simulink model "SG__MDL_IO344"  (R2020a)
settings: Solver=FixedStepAuto  StartTime=0.0  StopTime=Inf  RelTol=1e-3  EnableMultiTasking=on
model workspace (MAT data in the model file):
  a = 0.28
  ff = 1200
  fi = 150
  tmax = 40
libraries: dspfdesign x4, slrtlib x3, simulink x2, SG_library x1, dspsrcs4 x1
settings Model: SimulationMode=external  Creator=padlewsk  LastModifiedBy=padlewsk
settings SolverCC: ConcurrentTasks=on  AutoInsertRateTranBlk=on
settings DataIOCC: SaveFormat=StructureWithTime
settings OptimizationCC: BlockReduction=off  OptimizeBlockIOStorage=off
settings DebuggingCC: SFMachineParentedDataDiag=error
settings HardwareCC: ProdBitPerPointer=32  ProdBitPerSizeT=32  ProdBitPerPtrDiffT=32  ProdLargestAtomicFloat=None  ProdWordSize=32  ProdLongLongMode=on  ProdHWDeviceType=Generic->32-bit x86 compatible
settings RTWCC: Description=Simulink Real-Time  SystemTargetFile=slrt.tlc  TemplateMakefile=slrt_default_tmf  CodeExecutionProfiling=on  RTWCompilerOptimization=on
settings SimulinkRealTimeCC: SupportVariableSizeSignals=on  xPCConcurrentTasks=on

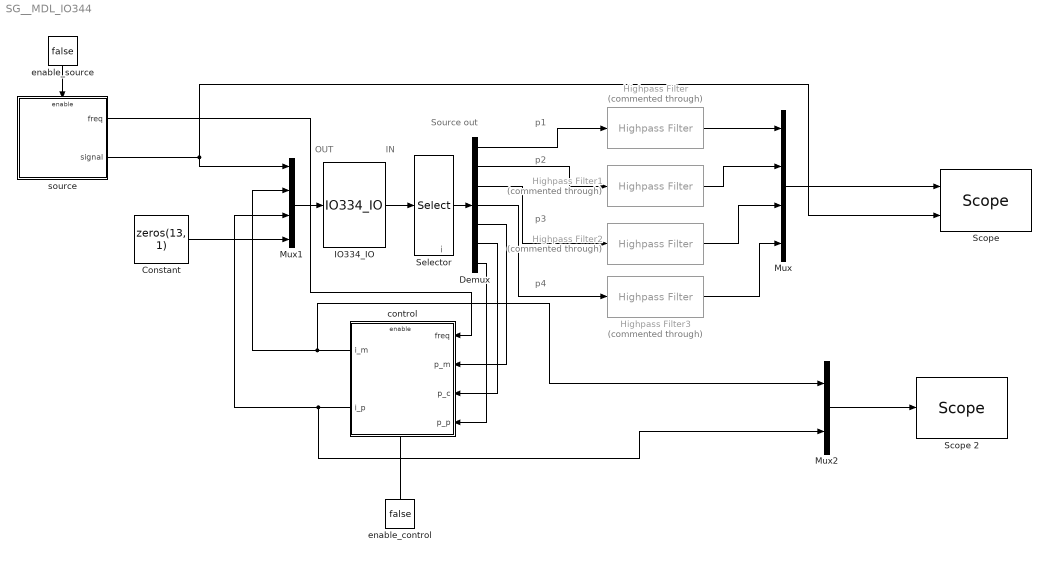
== system SG__MDL_IO344 ==
  note: p2
  note: i
  note: p3
  note: p1
  note: Source out
  note: IN
  note: OUT
  note: p4
  Constant : Constant  Value=zeros(13, 1)  SampleTime=-1
  Demux : Demux  Outputs=7
  Highpass Filter : dspfdesign/Highpass Filter  Commented=through  FilterType=IIR  DesignForMinimumOrder=off  FilterOrder=4  StopbandFrequency=8e3  PassbandFrequency=5  StopbandAttenuation=80  PassbandRipple=0.1  InheritSampleRate=off  SampleRate=65536  SimulateUsing=Interpreted execution  roundingMode=Floor  coeffsDataTypeStr=fixdt(1,16)
  Highpass Filter1 : dspfdesign/Highpass Filter  Commented=through  FilterType=IIR  DesignForMinimumOrder=off  FilterOrder=4  StopbandFrequency=8e3  PassbandFrequency=5  StopbandAttenuation=80  PassbandRipple=0.1  InheritSampleRate=off  SampleRate=65536  SimulateUsing=Interpreted execution  roundingMode=Floor  coeffsDataTypeStr=fixdt(1,16)
  Highpass Filter2 : dspfdesign/Highpass Filter  Commented=through  FilterType=IIR  DesignForMinimumOrder=off  FilterOrder=4  StopbandFrequency=8e3  PassbandFrequency=5  StopbandAttenuation=80  PassbandRipple=0.1  InheritSampleRate=off  SampleRate=65536  SimulateUsing=Interpreted execution  roundingMode=Floor  coeffsDataTypeStr=fixdt(1,16)
  Highpass Filter3 : dspfdesign/Highpass Filter  Commented=through  FilterType=IIR  DesignForMinimumOrder=off  FilterOrder=4  StopbandFrequency=4  PassbandFrequency=5  StopbandAttenuation=80  PassbandRipple=0.1  InheritSampleRate=off  SampleRate=65536  SimulateUsing=Interpreted execution  roundingMode=Floor  coeffsDataTypeStr=fixdt(1,16)
  IO334_IO : SG_library/Built elements/IO334_IO  ts=1.5259e-05  OutputRange=Auto (same as ADC)
      settings: SourceProductName=Custom Speedgoat implementations
  Mux : Mux
  Mux1 : Mux
  Mux2 : Mux  Inputs=2
  "Scope " : slrtlib/Displays and Logging/Scope   scopeno=2  scopetype=Host  autostart=on  viewmode=Graphical redraw  formatstr='%15.6f'  grid=on  ylimits=[0,0]  nosamples=1000  noprepostsamples=0  interleave=1  triggermode=Signal triggering  triggersignal=1  trigsignalfromport=on  triggerlevel=0.001  triggerslope=Either  triggerscope=1  triggersample=0  filename=data.dat  mode=Lazy  writesize=512  autorestart=off  dynamicfilemode=off  maxwritefilesize=512*1024^2
  Scope 2 : slrtlib/Displays and Logging/Scope   scopeno=3  scopetype=Target  autostart=on  viewmode=Graphical redraw  formatstr='%15.6f'  grid=on  ylimits=[0 0]  nosamples=250  noprepostsamples=0  interleave=1  triggermode=FreeRun  triggersignal=1  trigsignalfromport=off  triggerlevel=0.45  triggerslope=Either  triggerscope=1  triggersample=0  filename=data.dat  mode=Lazy  writesize=512  autorestart=off  dynamicfilemode=off  maxwritefilesize=512*1024^2
  Selector : Selector  InputPortWidth=16  IndexOptions=Index vector (dialog)  Indices=1:7  OutputSizes=1
  control : Subsystem
  enable_control : Constant  Value=false  SampleTime=-1
  enable_source : Constant  Value=false  SampleTime=-1
  source : Subsystem  TreatAsAtomicUnit=on
  wires:
  enable_source/1 -> source/Enable
  Mux/1 -> "Scope "/1
  Highpass Filter2/1 -> Mux/3
  Demux/1 -> Highpass Filter/1
  Highpass Filter/1 -> Mux/1
  Demux/3 -> Highpass Filter2/1
  Highpass Filter1/1 -> Mux/2
  Demux/4 -> Highpass Filter3/1
  IO334_IO/1 -> Selector/1
  Constant/1 -> Mux1/4
  Selector/1 -> Demux/1
  Demux/2 -> Highpass Filter1/1
  Mux1/1 -> IO334_IO/1
  source/1(freq) -> control/1(freq)
  Demux/5 -> control/2(p_m)
  control/2(i_p) -> Mux2/2, Mux1/3
  enable_control/1 -> control/Enable
  Demux/7 -> control/4(p_p)
  Demux/6 -> control/3(p_c)
  source/2(signal) -> Mux1/1, "Scope "/2
  Mux2/1 -> Scope 2/1
  Highpass Filter3/1 -> Mux/4
  control/1(i_m) -> Mux2/1, Mux1/2

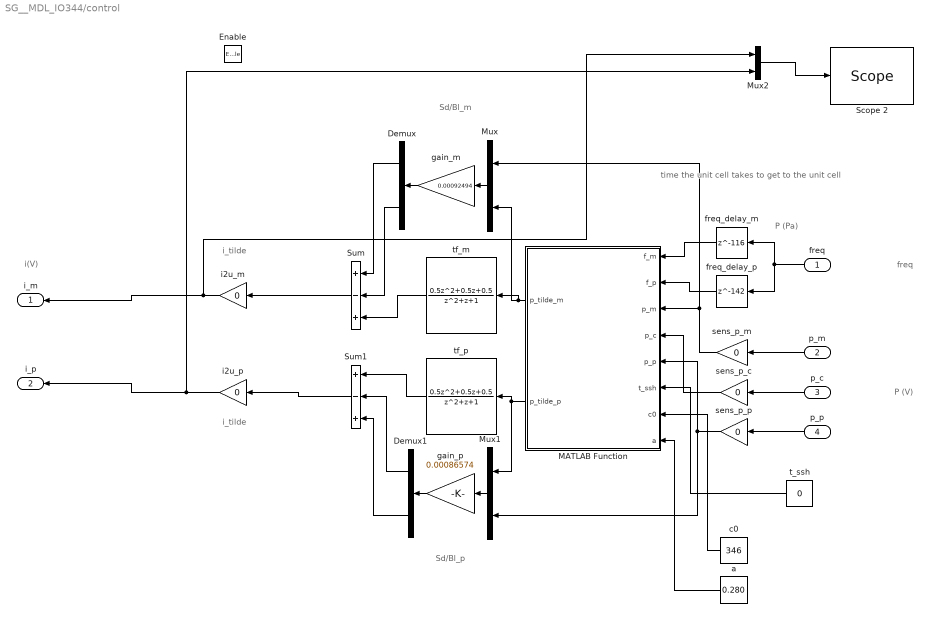
== system SG__MDL_IO344/control ==
  note: time the unit cell takes to get to the unit cell
  note: Sd/Bl_p
  note: P (Pa)
  note: P (V)
  note: i_tilde
  note: i(V)
  note: freq
  note: i_tilde
  note: Sd/Bl_m
  freq : Inport
  p_m : Inport  Port=2
  p_c : Inport  Port=3
  p_p : Inport  Port=4
  Enable : EnablePort
  Demux : Demux  Outputs=2
  Demux1 : Demux  Outputs=2
  MATLAB Function : MATLAB Function  TreatAsAtomicUnit=on
  Mux : Mux  Inputs=2
  Mux1 : Mux  Inputs=2
  Mux2 : Mux  Inputs=2
  Scope 2 : slrtlib/Displays and Logging/Scope   scopeno=1  scopetype=Target  autostart=on  viewmode=Graphical redraw  formatstr='%15.6f'  grid=on  ylimits=[0 0]  nosamples=250  noprepostsamples=0  interleave=1  triggermode=FreeRun  triggersignal=1  trigsignalfromport=off  triggerlevel=0.45  triggerslope=Either  triggerscope=1  triggersample=0  filename=data.dat  mode=Lazy  writesize=512  autorestart=off  dynamicfilemode=off  maxwritefilesize=512*1024^2
  Sum : Sum  Inputs=+-+
  Sum1 : Sum  Inputs=+-+
  a : Constant  Value=0.280
  c0 : Constant  Value=346
  freq_delay_m : Delay  DelayLength=116  InitialCondition=1
  freq_delay_p : Delay  DelayLength=142  InitialCondition=1
  gain_m : Gain  Gain=0.00092494
  gain_p : Gain  Gain=0.00086574
  i2u_m : Gain  Gain=0
  i2u_p : Gain  Gain=0
  sens_p_c : Gain  Gain=0
  sens_p_m : Gain  Gain=0
  sens_p_p : Gain  Gain=0
  t_ssh : Constant  Value=0
  tf_m : DiscreteTransferFcn  Numerator="[0.5         0.5         0.5]"  Denominator="[1  1  1]"
  tf_p : DiscreteTransferFcn  Numerator="[0.5         0.5         0.5]"  Denominator="[1  1  1]"
  i_m : Outport
  i_p : Outport  Port=2
  wires:
  p_m/1 -> sens_p_m/1
  sens_p_m/1 -> Mux/1, MATLAB Function/3(p_m)
  p_c/1 -> sens_p_c/1
  p_p/1 -> sens_p_p/1
  t_ssh/1 -> MATLAB Function/6(t_ssh)
  sens_p_c/1 -> MATLAB Function/4(p_c)
  sens_p_p/1 -> MATLAB Function/5(p_p), Mux1/2
  Demux1/1 -> Sum1/2
  Demux1/2 -> Sum1/3
  Demux/2 -> Sum/2
  Demux/1 -> Sum/1
  Mux/1 -> gain_m/1
  gain_m/1 -> Demux/1
  Mux1/1 -> gain_p/1
  gain_p/1 -> Demux1/1
  Mux2/1 -> Scope 2/1
  tf_m/1 -> Sum/3
  tf_p/1 -> Sum1/1
  freq/1 -> freq_delay_p/1, freq_delay_m/1
  i2u_p/1 -> Mux2/2, i_p/1
  freq_delay_m/1 -> MATLAB Function/1(f_m)
  i2u_m/1 -> Mux2/1, i_m/1
  freq_delay_p/1 -> MATLAB Function/2(f_p)
  c0/1 -> MATLAB Function/7(c0)
  a/1 -> MATLAB Function/8(a)
  MATLAB Function/2(p_tilde_p) -> Mux1/1, tf_p/1
  MATLAB Function/1(p_tilde_m) -> tf_m/1, Mux/2
  Sum/1 -> i2u_m/1
  Sum1/1 -> i2u_p/1

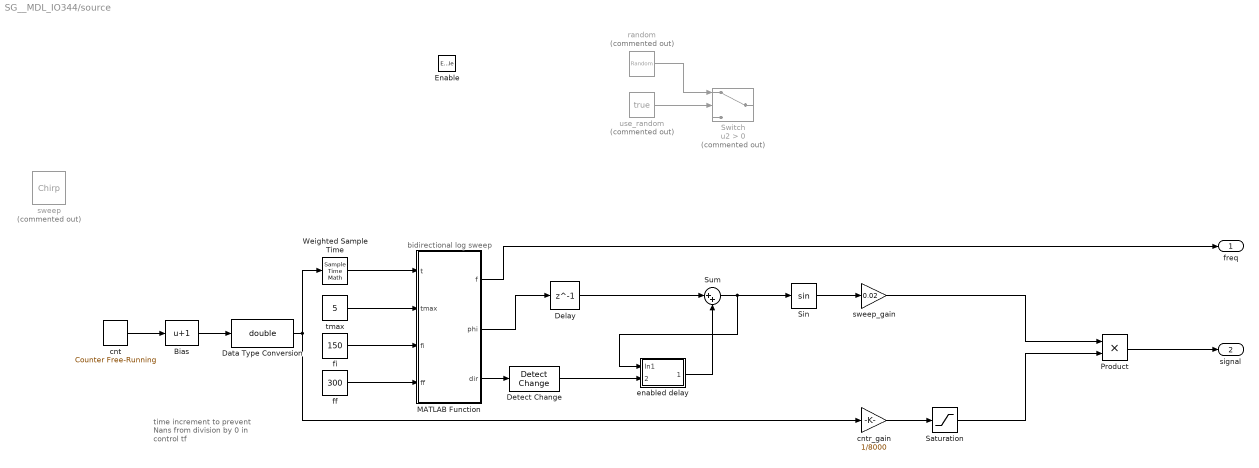
== system SG__MDL_IO344/source ==
  note: bidirectional log sweep
  note: time increment to prevent Nans from division by 0 in control tf
  Enable : EnablePort  StatesWhenEnabling=reset
  Bias : Bias  Bias=1
  Data Type Conversion : DataTypeConversion  OutDataTypeStr=double
  Delay : Delay  DelayLength=1
  Detect Change : simulink/Logic and Bit Operations/Detect Change  vinit=false  OutDataTypeStr=boolean
  MATLAB Function : MATLAB Function  TreatAsAtomicUnit=on
  Product : Product
  Saturation : Saturate  UpperLimit=1  LowerLimit=0
  Sin : Trigonometry
  Sum : Sum  Inputs=|++
  Switch : Switch  Commented=on  Criteria=u2 > Threshold
  Weighted Sample Time : SampleTimeMath  TsampMathOp=*
  cnt : simulink/Sources/Counter Free-Running  NumBits=32  tsamp=1.5259e-05
  cntr_gain : Gain  Gain=1/8000  ParamDataTypeStr=double
  enabled delay : Subsystem
  ff : Constant  Value=300
  fi : Constant  Value=150
  random : RandomNumber  Commented=on  Variance=0.5  SampleTime=3.5e-05
  sweep : dspsrcs4/Chirp  Commented=on  sweep=Logarithmic  mode=Bidirectional  f0=150  f1=1200  t1=10  Tsweep=20  phase=0  Ts=3.5e-05  spf=1  datatype=Double  OutputFrames=off
  sweep_gain : Gain  Gain=0.02
  tmax : Constant  Value=5
  use_random : Constant  Commented=on  Value=true  SampleTime=-1
  freq : Outport  OutputWhenDisabled=reset  InitialOutput=0  VectorParamsAs1DForOutWhenUnconnected=off
  signal : Outport  Port=2  OutputWhenDisabled=reset  InitialOutput=0  VectorParamsAs1DForOutWhenUnconnected=off
  wires:
  use_random/1 -> Switch/2
  random/1 -> Switch/1
  sweep_gain/1 -> Product/1
  cntr_gain/1 -> Saturation/1
  Product/1 -> signal/1
  MATLAB Function/2(phi) -> Delay/1
  Saturation/1 -> Product/2
  Weighted Sample Time/1 -> MATLAB Function/1(t)
  Data Type Conversion/1 -> cntr_gain/1, Weighted Sample Time/1
  MATLAB Function/1(f) -> freq/1
  Sin/1 -> sweep_gain/1
  MATLAB Function/3(dir) -> Detect Change/1
  Detect Change/1 -> enabled delay/2(enable)
  Delay/1 -> Sum/1
  enabled delay/1(Out1) -> Sum/2
  Sum/1 -> enabled delay/1(In1), Sin/1
  cnt/1 -> Bias/1
  Bias/1 -> Data Type Conversion/1
  ff/1 -> MATLAB Function/4(ff)
  tmax/1 -> MATLAB Function/2(tmax)
  fi/1 -> MATLAB Function/3(fi)

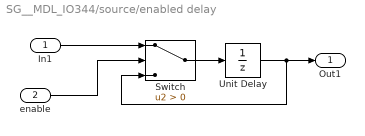
== system SG__MDL_IO344/source/enabled delay ==
  In1 : Inport
  enable : Inport  Port=2
  Switch : Switch  Criteria=u2 > Threshold
  Unit Delay : UnitDelay  SampleTime=-1  HasFrameUpgradeWarning=on
  Out1 : Outport
  wires:
  Unit Delay/1 -> Switch/3, Out1/1
  Switch/1 -> Unit Delay/1
  In1/1 -> Switch/1
  enable/1 -> Switch/2

== matlab function SG__MDL_IO344/control/MATLAB Function ==
  data: f_m input; f_p input; p_tilde_m output; p_m input; p_c input; p_p input; t_ssh input; p_tilde_p output; c0 input; a input
function [p_tilde_m, p_tilde_p] = p_tilde(f_m,f_p,p_m,p_c,p_p, t_ssh, c0, a)%frequency and pressure
% c0 and a are set as parameters and directly read from the workspace 
k_m = 2*pi*f_m/c0 %corresponding wave vector%%
k_p = 2*pi*f_p/c0 %corresponding wave vector%%

p_tilde_m = (p_m*sin(k_m*a*(t_ssh-1)/4) + p_c*sin(-k_m*a*t_ssh/4))/sin(-k_m*a/4) ;
p_tilde_p = (p_p*sin(-k_p*a*(t_ssh-1)/4) + p_c*sin(k_p*a*t_ssh/4))/sin(k_p*a/4) ;

%p_tilde_m = (p_c);
%p_tilde_p = (p_c);

== matlab function SG__MDL_IO344/source/MATLAB Function ==
  data: f output; t input; tmax input; phi output; dir output; fi input; ff input
function [f, phi, dir] = fcn(t, tmax, fi, ff)
%tmax is the time at which the maximum frequency is reached

t = mod(t, 2*tmax);

if t < tmax
    % up
    dir = 1;
    
    
    % linear (CF wikipedia)
%     phi = 2*pi*(0.5*(ff - fi)*t^2/tmax + fi*t);
%     f = fi + (ff - fi)*t/tmax;
    
    % logarithmic %%% https://en.wikipedia.org/wiki/Chirp
    k = log((ff/fi)^(1/tmax));
    phi = 2*pi*fi*(exp(k*t) - 1)/k;
    f = fi*exp(k*t);
else
    % down
    dir = -1;
    
    
    % linear (CF wikipedia)
%     phi = 2*pi*(0.5*(fi - ff)*(t-tmax)^2/tmax + ff*(t-tmax)); % linear
%     f = ff + (fi - ff)*(t - tmax)/tmax;
    
    % logarithmic
    k = log((fi/ff)^(1/tmax));
    phi = 2*pi*ff*(exp(k*(t - tmax)) - 1)/k;
    f = ff*exp(k*(t-tmax));
end

phi = mod(phi, 2*pi);
